simulink model "impulse_response"  (R2025a)
settings: Solver=VariableStepAuto  StartTime=0.0  StopTime=3  RelTol=1e-3
libraries: SignalEditorBlockLib x1
settings Model: Creator=Имя  LastModifiedBy=Имя

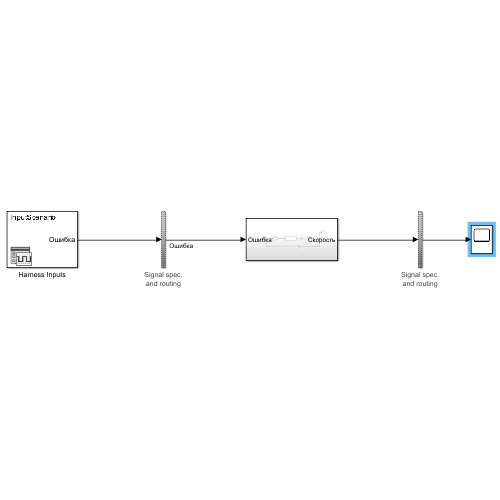
[thumbnail: Simulink's stored preview of the top-level diagram]
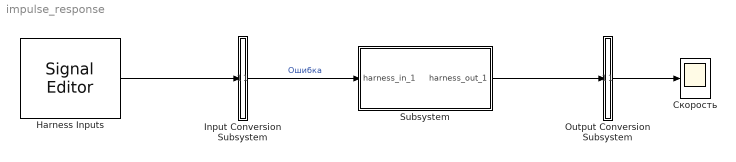
== system impulse_response ==
  Harness Inputs : SignalEditorBlockLib/Signal Editor  FileName=impulse_response_HarnessInputs.mat  ActiveScenario=InputScenario  ActiveSignal=Ошибка  IsBus=off  OutputBusObjectStr=Bus: BusObject  SampleTime=0  Interpolate=off  ZeroCross=off  OutputAfterFinalValue=Setting to zero  Unit=inherit  PreserveSignalName=on  ApplySigPropsToAllScenarios=on  ApplySigPropsToAllSignals=off  SignalPropertySource=Dialog parameters
  Input Conversion Subsystem : Subsystem  Tag=__SLT_ICS__  Description=|
      | Signal spec.
      | and routing
      settings: AttributesFormatString=%<Description>
  Output Conversion Subsystem : Subsystem  Tag=__SLT_OCS__  Description=|
      | Signal spec.
      | and routing
      settings: AttributesFormatString=%<Description>
  Subsystem : Subsystem  Tag=__SL_testing_harness_stub_
  Скорость : Scope
      settings: ActiveDisplayYMinimum=-100  ActiveDisplayYMaximum=1000
  wires:
  Harness Inputs/1 -> Input Conversion Subsystem/1(Inport_1)
  Output Conversion Subsystem/1(Outport_1) -> Скорость/1
  Input Conversion Subsystem/1(Outport_1) -> Subsystem/1(harness_in_1)  "Ошибка"
  Subsystem/1(harness_out_1) -> Output Conversion Subsystem/1(Inport_1)

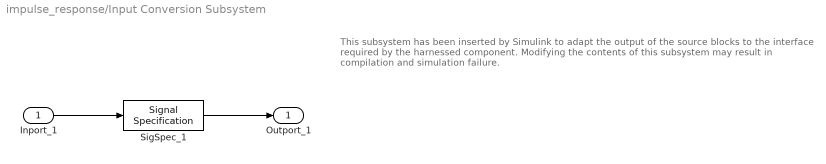
== system impulse_response/Input Conversion Subsystem ==
  note: This subsystem has been inserted by Simulink to adapt the output of the source blocks to the interface required by the harnessed component.
      |  Modifying the contents of this subsystem may result in compilation and simulation failure.
  Inport_1 : Inport
  SigSpec_1 : SignalSpecification  OutDataTypeStr=double  Dimensions=[1]  SampleTime=[0, 0]
  Outport_1 : Outport
  wires:
  SigSpec_1/1 -> Outport_1/1
  Inport_1/1 -> SigSpec_1/1

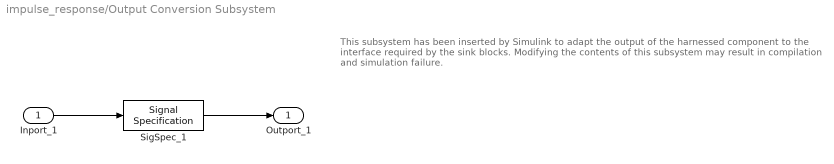
== system impulse_response/Output Conversion Subsystem ==
  note: This subsystem has been inserted by Simulink to adapt the output of the harnessed component to the interface required by the sink blocks.
      |  Modifying the contents of this subsystem may result in compilation and simulation failure.
  Inport_1 : Inport
  SigSpec_1 : SignalSpecification  OutDataTypeStr=double  Dimensions=[1]
  Outport_1 : Outport
  wires:
  Inport_1/1 -> SigSpec_1/1
  SigSpec_1/1 -> Outport_1/1

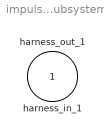
== system impulse_response/Subsystem ==
  harness_in_1 : Inport
  harness_out_1 : Outport
